simulink model "SIMULINK_U_f_C"  (R2018b)
settings: Solver=FixedStepAuto  StartTime=0.0  StopTime=sim_end_time  FixedStep=fixed_step_size  RelTol=1e-3
undefined symbols (not defined in the file): a, act_end, b, battery_threshold, bb, draw_gif, droneyeeUAV2_NUM, droneyeeUAV3_NUM, droneyeeUAV4_NUM, droneyeeUAV5_NUM, fixed_step_size, k, KD_x, KD_y, kd_z, KDD_x, KDD_y, KI_x, KI_y, ki_z, KII_x, KII_y, KP_x, KP_y, kp_z, KPP_x, KPP_y, lmt, omega, R, sim_end_time, uav10num, uav1num, uav2num, uav3num, uav4num, uav5num, uav6num, uav7num, uav8num, uav9num, UAV_NUM, Vel_Switch_1, Vel_Switch_10, Vel_Switch_11, Vel_Switch_12, Vel_Switch_13, Vel_Switch_14, Vel_Switch_15, Vel_Switch_16, Vel_Switch_17, Vel_Switch_18, Vel_Switch_19, Vel_Switch_2, Vel_Switch_20, Vel_Switch_3, Vel_Switch_4, Vel_Switch_5, Vel_Switch_6, Vel_Switch_7 ... (+11)
libraries: simulink x120, aerolibanimutils x1
(part 2 of 10)

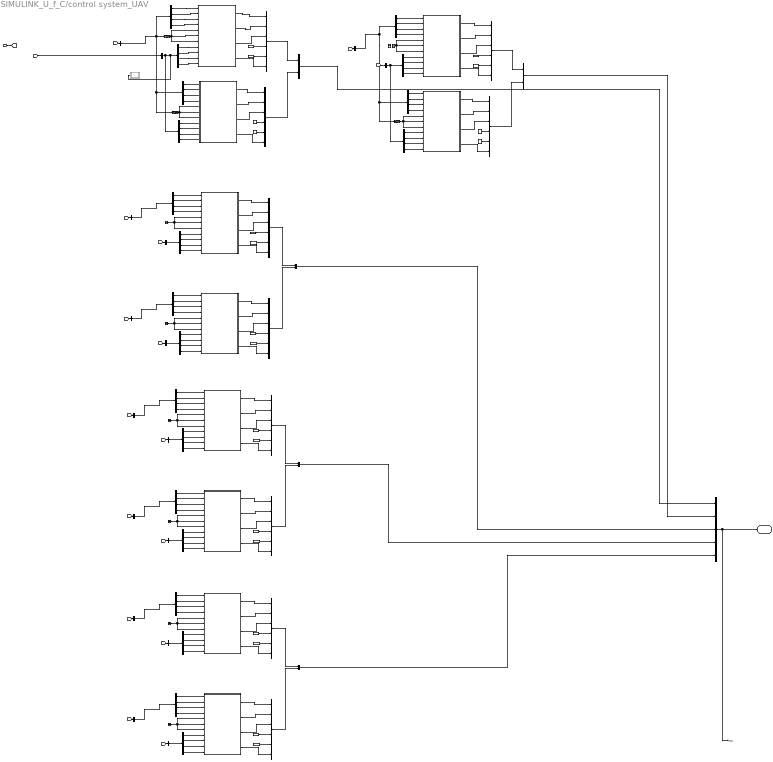
== system SIMULINK_U_f_C/control system_UAV ==
  uavstates_d : Inport
  Baseline Controller1 : Subsystem  AncestorBlock=ARBlocks/Baseline Controller
  Baseline Controller10 : Subsystem  AncestorBlock=ARBlocks/Baseline Controller
  Baseline Controller2 : Subsystem  AncestorBlock=ARBlocks/Baseline Controller
  Baseline Controller3 : Subsystem  AncestorBlock=ARBlocks/Baseline Controller
  Baseline Controller4 : Subsystem  AncestorBlock=ARBlocks/Baseline Controller
  Baseline Controller5 : Subsystem  AncestorBlock=ARBlocks/Baseline Controller
  Baseline Controller6 : Subsystem  AncestorBlock=ARBlocks/Baseline Controller
  Baseline Controller7 : Subsystem  AncestorBlock=ARBlocks/Baseline Controller
  Baseline Controller8 : Subsystem  AncestorBlock=ARBlocks/Baseline Controller
  Baseline Controller9 : Subsystem  AncestorBlock=ARBlocks/Baseline Controller
  Bus Creator{,1,3..4,6..7,9..10,12,14} (10 alike) : BusCreator  Inputs=6
  Bus Creator{2,5,8,11,13} (5 alike) : BusCreator  Inputs=2
  Bus Creator36 : BusCreator  Inputs=5
  Bus Selector : BusSelector  OutputSignals=droneyeeUAV1_states,droneyeeUAV2_states  OutputAsBus=on
  Bus Selector1 : BusSelector  OutputSignals=droneyeeUAV1_d.x1_d,droneyeeUAV1_d.y1_d,droneyeeUAV1_d.z1_d,droneyeeUAV1_d.yaw1_d
  Bus Selector10 : BusSelector  OutputSignals=droneyeeUAV4_d.x4_d,droneyeeUAV4_d.y4_d,droneyeeUAV4_d.z4_d,droneyeeUAV4_d.yaw4_d
  Bus Selector11 : BusSelector  OutputSignals=states_5_6_d
  Bus Selector12 : BusSelector  OutputSignals=droneyeeUAV3_states.x,droneyeeUAV3_states.y,droneyeeUAV3_states.z,droneyeeUAV3_states.yaw
  Bus Selector13 : BusSelector  OutputSignals=droneyeeUAV5_d.x5_d,droneyeeUAV5_d.y5_d,droneyeeUAV5_d.z5_d,droneyeeUAV5_d.yaw5_d
  Bus Selector14 : BusSelector  OutputSignals=states_7_8_d.droneyeeUAV8_d
  Bus Selector{15..16,24..25} (4 alike) : BusSelector  OutputSignals=x_d,y_d,z_d,yaw_d
  Bus Selector{6,17,20,23,26,29} (6 alike) : BusSelector  OutputSignals=x,y,z,yaw
  Bus Selector18 : BusSelector  OutputSignals=droneyeeUAV7_states
  Bus Selector19 : BusSelector  OutputSignals=states_7_8_d.droneyeeUAV7_d
  Bus Selector2 : BusSelector  OutputSignals=droneyeeUAV6_d.x_d,droneyeeUAV6_d.y_d,droneyeeUAV6_d.z_d,droneyeeUAV6_d.yaw_d
  Bus Selector21 : BusSelector  OutputSignals=droneyeeUAV8_states
  Bus Selector22 : BusSelector  OutputSignals=states_9_10_d.droneyeeUAV10_d
  Bus Selector27 : BusSelector  OutputSignals=droneyeeUAV9_states
  Bus Selector28 : BusSelector  OutputSignals=states_9_10_d.droneyeeUAV9_d
  Bus Selector3 : BusSelector  OutputSignals=droneyeeUAV2_states.x,droneyeeUAV2_states.y,droneyeeUAV2_states.z,droneyeeUAV2_states.yaw
  Bus Selector30 : BusSelector  OutputSignals=droneyeeUAV10_states
  Bus Selector31 : BusSelector  OutputSignals=droneyeeUAV3_states,droneyeeUAV4_states  OutputAsBus=on
  Bus Selector32 : BusSelector  OutputSignals=droneyeeUAV5_states
  Bus Selector37 : BusSelector  OutputSignals=states_5_6_d
  Bus Selector38 : BusSelector  OutputSignals=states1_2_d
  Bus Selector39 : BusSelector  OutputSignals=states_3_4_d
  Bus Selector4 : BusSelector  OutputSignals=droneyeeUAV2_d.x2_d,droneyeeUAV2_d.y2_d,droneyeeUAV2_d.z2_d,droneyeeUAV2_d.yaw2_d
  Bus Selector5 : BusSelector  OutputSignals=droneyeeUAV3_d.x3_d,droneyeeUAV3_d.y3_d,droneyeeUAV3_d.z3_d,droneyeeUAV3_d.yaw3_d
  Bus Selector7 : BusSelector  OutputSignals=droneyeeUAV6_states
  Bus Selector8 : BusSelector  OutputSignals=droneyeeUAV1_states.x,droneyeeUAV1_states.y,droneyeeUAV1_states.z,droneyeeUAV1_states.yaw
  Bus Selector9 : BusSelector  OutputSignals=droneyeeUAV4_states.x,droneyeeUAV4_states.y,droneyeeUAV4_states.z,droneyeeUAV4_states.yaw
  Constant{,1..19} (20 alike) : Constant  Value=0
  Goto : Goto  Commented=on  GotoTag=uav_ctrl  TagVisibility=global
  Ground{,1..9} (10 alike) : Ground
  MATLAB Function : MATLAB Function  Commented=on  TreatAsAtomicUnit=on
  Terminator{,1..3} (4 alike) : Terminator
  uav_ctrl : Outport
  tag scope: uav1_24_d=global
  wires:
  Bus Selector1/2 -> Baseline Controller1/9(y_d)  "<y1_d>"
  Bus Selector8/3 -> Baseline Controller1/3(" Z_e ")  "<z>"
  Bus Selector1/3 -> Baseline Controller1/10(Z_d)  "<z1_d>"
  Bus Selector8/4 -> Baseline Controller1/4(Yaw_e)  "<yaw>"
  Bus Selector3/4 -> Baseline Controller2/4(Yaw_e)  "<yaw>"
  Bus Selector3/2 -> Baseline Controller2/2(Y_e)  "<y>"
  Bus Selector1/1 -> Baseline Controller1/8(x_d)  "<x1_d>"
  Bus Selector3/1 -> Baseline Controller2/1(X_e)  "<x>"
  Ground2/1 -> Baseline Controller2/7("V_z "), Baseline Controller2/5(" V_x"), Baseline Controller2/6(V_y)
  Bus Selector8/1 -> Baseline Controller1/1(X_e)  "<x>"
  Bus Selector3/3 -> Baseline Controller2/3(" Z_e ")  "<z>"
  Bus Selector1/4 -> Baseline Controller1/11(Yaw_d)  "<yaw1_d>"
  Bus Selector8/2 -> Baseline Controller1/2(Y_e)  "<y>"
  Ground1/1 -> Baseline Controller1/5(" V_x"), Baseline Controller1/6(V_y), Baseline Controller1/7("V_z ")
  Baseline Controller1/1(ux) -> Bus Creator/1  "u_vx"
  Baseline Controller1/2(uy) -> Bus Creator/2  "u_vy"
  Baseline Controller1/3(Z_velocity_d. [-1,1]) -> Bus Creator/3  "u_vz"
  Baseline Controller1/4(yaw_rate_d [-1,1]) -> Bus Creator/6  "u_rate_yaw"
  Constant/1 -> Bus Creator/4  "u_rate_roll"
  Constant1/1 -> Bus Creator/5  "u_rate_pitch"
  Baseline Controller2/4(yaw_rate_d [-1,1]) -> Bus Creator1/6  "u_rate_yaw"
  Baseline Controller2/1(ux) -> Bus Creator1/1  "u_vx"
  Constant2/1 -> Bus Creator1/4  "u_rate_roll"
  Baseline Controller2/2(uy) -> Bus Creator1/2  "u_vy"
  Baseline Controller2/3(Z_velocity_d. [-1,1]) -> Bus Creator1/3  "u_vz"
  Constant3/1 -> Bus Creator1/5  "u_rate_pitch"
  Bus Creator/1 -> Bus Creator2/1  "uav1"
  Bus Creator1/1 -> Bus Creator2/2  "uav2"
  Bus Creator2/1 -> Bus Creator36/1  "ctrl_1_2"
  Bus Selector38/1 -> Bus Selector4/1, MATLAB Function/1(u), Bus Selector1/1  "<states1_2_d>"
  Bus Selector4/1 -> Baseline Controller2/8(x_d)  "<x2_d>"
  Bus Selector4/3 -> Baseline Controller2/10(Z_d)  "<z2_d>"
  Bus Selector4/2 -> Baseline Controller2/9(y_d)  "<y2_d>"
  Bus Selector4/4 -> Baseline Controller2/11(Yaw_d)  "<yaw2_d>"
  Ground/1 -> Baseline Controller4/7("V_z "), Baseline Controller4/5(" V_x"), Baseline Controller4/6(V_y)
  Bus Selector12/4 -> Baseline Controller3/4(Yaw_e)  "<yaw>"
  Constant4/1 -> Bus Creator3/4  "u_rate_roll"
  Baseline Controller4/3(Z_velocity_d. [-1,1]) -> Bus Creator4/3  "u_vz"
  Baseline Controller3/3(Z_velocity_d. [-1,1]) -> Bus Creator3/3  "u_vz"
  Bus Selector5/4 -> Baseline Controller3/11(Yaw_d)  "<yaw3_d>"
  Baseline Controller4/1(ux) -> Bus Creator4/1  "u_vx"
  Bus Selector10/1 -> Baseline Controller4/8(x_d)  "<x4_d>"
  Bus Selector12/2 -> Baseline Controller3/2(Y_e)  "<y>"
  Baseline Controller4/4(yaw_rate_d [-1,1]) -> Bus Creator4/6  "u_rate_yaw"
  Bus Selector5/3 -> Baseline Controller3/10(Z_d)  "<z3_d>"
  Ground3/1 -> Baseline Controller3/7("V_z "), Baseline Controller3/5(" V_x"), Baseline Controller3/6(V_y)
  Bus Selector12/1 -> Baseline Controller3/1(X_e)  "<x>"
  Bus Selector10/2 -> Baseline Controller4/9(y_d)  "<y4_d>"
  Bus Selector9/4 -> Baseline Controller4/4(Yaw_e)  "<yaw>"
  Bus Selector12/3 -> Baseline Controller3/3(" Z_e ")  "<z>"
  Baseline Controller4/2(uy) -> Bus Creator4/2  "u_vy"
  Constant7/1 -> Bus Creator4/5  "u_rate_pitch"
  Baseline Controller3/1(ux) -> Bus Creator3/1  "u_vx"
  Bus Selector9/1 -> Baseline Controller4/1(X_e)  "<x>"
  Bus Selector5/2 -> Baseline Controller3/9(y_d)  "<y3_d>"
  Bus Selector39/1 -> Bus Selector10/1, Bus Selector5/1  "<states_3_4_d>"
  Bus Selector10/4 -> Baseline Controller4/11(Yaw_d)  "<yaw4_d>"
  Constant5/1 -> Bus Creator3/5  "u_rate_pitch"
  Bus Selector5/1 -> Baseline Controller3/8(x_d)  "<x3_d>"
  Constant6/1 -> Bus Creator4/4  "u_rate_roll"
  Bus Creator5/1 -> Bus Creator36/2  "ctrl_3_4"
  Bus Selector10/3 -> Baseline Controller4/10(Z_d)  "<z4_d>"
  Bus Selector9/2 -> Baseline Controller4/2(Y_e)  "<y>"
  Bus Creator3/1 -> Bus Creator5/1  "uav3"
  Bus Selector9/3 -> Baseline Controller4/3(" Z_e ")  "<z>"
  Baseline Controller3/4(yaw_rate_d [-1,1]) -> Bus Creator3/6  "u_rate_yaw"
  Baseline Controller3/2(uy) -> Bus Creator3/2  "u_vy"
  Bus Creator4/1 -> Bus Creator5/2  "uav4"
  Bus Selector23/2 -> Baseline Controller5/2(Y_e)  "<y>"
  Baseline Controller5/1(ux) -> Bus Creator6/1  "u_vx"
  Bus Selector13/4 -> Baseline Controller5/11(Yaw_d)  "<yaw5_d>"
  Bus Selector37/1 -> Bus Selector13/1  "<states_5_6_d>"
  Bus Selector13/2 -> Baseline Controller5/9(y_d)  "<y5_d>"
  Bus Selector23/1 -> Baseline Controller5/1(X_e)  "<x>"
  Constant8/1 -> Bus Creator6/4  "u_rate_roll"
  Bus Selector23/3 -> Baseline Controller5/3(" Z_e ")  "<z>"
  Bus Selector13/3 -> Baseline Controller5/10(Z_d)  "<z5_d>"
  Bus Selector23/4 -> Baseline Controller5/4(Yaw_e)  "<yaw>"
  Ground4/1 -> Baseline Controller5/7("V_z "), Baseline Controller5/5(" V_x"), Baseline Controller5/6(V_y)
  Bus Creator8/1 -> Bus Creator36/3  "ctrl_5_6"
  Baseline Controller5/3(Z_velocity_d. [-1,1]) -> Bus Creator6/3  "u_vz"
  Constant9/1 -> Bus Creator6/5  "u_rate_pitch"
  Bus Selector13/1 -> Baseline Controller5/8(x_d)  "<x5_d>"
  Baseline Controller5/4(yaw_rate_d [-1,1]) -> Bus Creator6/6  "u_rate_yaw"
  Baseline Controller5/2(uy) -> Bus Creator6/2  "u_vy"
  Bus Selector31/1 -> Bus Selector12/1, Terminator/1, Bus Selector9/1
  Bus Selector32/1 -> Bus Selector23/1  "<droneyeeUAV5_states>"
  [uav_states] -> Bus Selector/1
  Bus Selector/1 -> Terminator1/1, Terminator2/1, Bus Selector3/1, Bus Selector8/1
  [uav_states] -> Bus Selector31/1
  [uav_states] -> Bus Selector32/1
  [uav1_24_d] -> Bus Selector37/1
  [uav1_24_d] -> Bus Selector38/1
  [uav1_24_d] -> Bus Selector39/1
  Bus Creator36/1 -> Goto/1, uav_ctrl/1
  uavstates_d/1 -> [uav1_24_d]
  Bus Selector2/2 -> Baseline Controller6/9(y_d)  "<y_d>"
  Bus Selector6/3 -> Baseline Controller6/3(" Z_e ")  "<z>"
  Baseline Controller6/4(yaw_rate_d [-1,1]) -> Bus Creator7/6  "u_rate_yaw"
  Constant11/1 -> Bus Creator7/5  "u_rate_pitch"
  Baseline Controller6/1(ux) -> Bus Creator7/1  "u_vx"
  Bus Selector2/4 -> Baseline Controller6/11(Yaw_d)  "<yaw_d>"
  Constant10/1 -> Bus Creator7/4  "u_rate_roll"
  Bus Selector6/2 -> Baseline Controller6/2(Y_e)  "<y>"
  Ground5/1 -> Baseline Controller6/7("V_z "), Baseline Controller6/5(" V_x"), Baseline Controller6/6(V_y)
  Bus Selector7/1 -> Bus Selector6/1  "<droneyeeUAV6_states>"
  Bus Selector6/1 -> Baseline Controller6/1(X_e)  "<x>"
  Bus Selector2/1 -> Baseline Controller6/8(x_d)  "<x_d>"
  Baseline Controller6/2(uy) -> Bus Creator7/2  "u_vy"
  Bus Selector6/4 -> Baseline Controller6/4(Yaw_e)  "<yaw>"
  [uav1_24_d] -> Bus Selector11/1
  Bus Selector11/1 -> Bus Selector2/1  "<states_5_6_d>"
  Baseline Controller6/3(Z_velocity_d. [-1,1]) -> Bus Creator7/3  "u_vz"
  Bus Selector2/3 -> Baseline Controller6/10(Z_d)  "<z_d>"
  [uav_states] -> Bus Selector7/1
  Bus Creator6/1 -> Bus Creator8/1  "ctrl_5"
  Bus Creator7/1 -> Bus Creator8/2  "ctrl_5"
  Bus Selector15/2 -> Baseline Controller7/9(y_d)  "<y_d>"
  [uav_states] -> Bus Selector21/1
  Baseline Controller8/2(uy) -> Bus Creator10/2  "u_vy"
  Bus Selector21/1 -> Bus Selector20/1  "<droneyeeUAV8_states>"
  Bus Selector14/1 -> Bus Selector16/1  "<droneyeeUAV8_d>"
  Bus Selector16/1 -> Baseline Controller8/8(x_d)  "<x_d>"
  Bus Selector20/2 -> Baseline Controller8/2(Y_e)  "<y>"
  Bus Selector20/1 -> Baseline Controller8/1(X_e)  "<x>"
  Ground7/1 -> Baseline Controller8/7("V_z "), Baseline Controller8/5(" V_x"), Baseline Controller8/6(V_y)
  Bus Selector16/4 -> Baseline Controller8/11(Yaw_d)  "<yaw_d>"
  Constant13/1 -> Bus Creator10/5  "u_rate_pitch"
  Bus Selector20/4 -> Baseline Controller8/4(Yaw_e)  "<yaw>"
  Baseline Controller8/4(yaw_rate_d [-1,1]) -> Bus Creator10/6  "u_rate_yaw"
  Bus Selector17/3 -> Baseline Controller7/3(" Z_e ")  "<z>"
  Bus Selector16/2 -> Baseline Controller8/9(y_d)  "<y_d>"
  Baseline Controller7/4(yaw_rate_d [-1,1]) -> Bus Creator9/6  "u_rate_yaw"
  Constant15/1 -> Bus Creator9/5  "u_rate_pitch"
  Bus Selector20/3 -> Baseline Controller8/3(" Z_e ")  "<z>"
  Bus Selector16/3 -> Baseline Controller8/10(Z_d)  "<z_d>"
  Baseline Controller7/1(ux) -> Bus Creator9/1  "u_vx"
  Bus Selector15/4 -> Baseline Controller7/11(Yaw_d)  "<yaw_d>"
  Constant14/1 -> Bus Creator9/4  "u_rate_roll"
  Baseline Controller8/3(Z_velocity_d. [-1,1]) -> Bus Creator10/3  "u_vz"
  Baseline Controller8/1(ux) -> Bus Creator10/1  "u_vx"
  Bus Selector17/2 -> Baseline Controller7/2(Y_e)  "<y>"
  Ground6/1 -> Baseline Controller7/7("V_z "), Baseline Controller7/5(" V_x"), Baseline Controller7/6(V_y)
  Bus Selector18/1 -> Bus Selector17/1  "<droneyeeUAV7_states>"
  Bus Selector17/1 -> Baseline Controller7/1(X_e)  "<x>"
  Bus Selector15/1 -> Baseline Controller7/8(x_d)  "<x_d>"
  Baseline Controller7/2(uy) -> Bus Creator9/2  "u_vy"
  Bus Creator10/1 -> Bus Creator11/2  "ctrl_5"
  Bus Selector17/4 -> Baseline Controller7/4(Yaw_e)  "<yaw>"
  Constant12/1 -> Bus Creator10/4  "u_rate_roll"
  [uav1_24_d] -> Bus Selector19/1
  [uav1_24_d] -> Bus Selector14/1
  Bus Selector19/1 -> Bus Selector15/1  "<droneyeeUAV7_d>"
  Baseline Controller7/3(Z_velocity_d. [-1,1]) -> Bus Creator9/3  "u_vz"
  Bus Selector15/3 -> Baseline Controller7/10(Z_d)  "<z_d>"
  [uav_states] -> Bus Selector18/1
  Bus Creator9/1 -> Bus Creator11/1  "ctrl_5"
  Bus Creator11/1 -> Bus Creator36/4  "ctrl_7_8"
  Bus Creator12/1 -> Bus Creator13/2  "ctrl_5"
  Bus Selector26/1 -> Baseline Controller9/1(X_e)  "<x>"
  Bus Selector24/1 -> Baseline Controller9/8(x_d)  "<x_d>"
  Bus Selector27/1 -> Bus Selector26/1  "<droneyeeUAV9_states>"
  Ground8/1 -> Baseline Controller9/7("V_z "), Baseline Controller9/5(" V_x"), Baseline Controller9/6(V_y)
  Baseline Controller10/1(ux) -> Bus Creator12/1  "u_vx"
  Baseline Controller9/2(uy) -> Bus Creator14/2  "u_vy"
  Bus Selector25/3 -> Baseline Controller10/10(Z_d)  "<z_d>"
  Bus Selector24/4 -> Baseline Controller9/11(Yaw_d)  "<yaw_d>"
  Constant18/1 -> Bus Creator14/4  "u_rate_roll"
  Bus Selector29/3 -> Baseline Controller10/3(" Z_e ")  "<z>"
  Baseline Controller9/4(yaw_rate_d [-1,1]) -> Bus Creator14/6  "u_rate_yaw"
  Constant19/1 -> Bus Creator14/5  "u_rate_pitch"
  Bus Selector26/3 -> Baseline Controller9/3(" Z_e ")  "<z>"
  Bus Selector25/2 -> Baseline Controller10/9(y_d)  "<y_d>"
  Baseline Controller10/4(yaw_rate_d [-1,1]) -> Bus Creator12/6  "u_rate_yaw"
  Bus Selector29/4 -> Baseline Controller10/4(Yaw_e)  "<yaw>"
  Ground9/1 -> Baseline Controller10/7("V_z "), Baseline Controller10/5(" V_x"), Baseline Controller10/6(V_y)
  Bus Selector25/4 -> Baseline Controller10/11(Yaw_d)  "<yaw_d>"
  Bus Selector29/1 -> Baseline Controller10/1(X_e)  "<x>"
  Baseline Controller10/3(Z_velocity_d. [-1,1]) -> Bus Creator12/3  "u_vz"
  Bus Selector29/2 -> Baseline Controller10/2(Y_e)  "<y>"
  Bus Selector25/1 -> Baseline Controller10/8(x_d)  "<x_d>"
  Bus Selector30/1 -> Bus Selector29/1  "<droneyeeUAV10_states>"
  Bus Selector22/1 -> Bus Selector25/1  "<droneyeeUAV10_d>"
  [uav_states] -> Bus Selector30/1
  Baseline Controller10/2(uy) -> Bus Creator12/2  "u_vy"
  Bus Selector24/2 -> Baseline Controller9/9(y_d)  "<y_d>"
  Bus Selector24/3 -> Baseline Controller9/10(Z_d)  "<z_d>"
  Bus Creator14/1 -> Bus Creator13/1  "ctrl_5"
  [uav1_24_d] -> Bus Selector28/1
  [uav_states] -> Bus Selector27/1
  Constant17/1 -> Bus Creator12/5  "u_rate_pitch"
  Bus Selector26/4 -> Baseline Controller9/4(Yaw_e)  "<yaw>"
  Bus Selector26/2 -> Baseline Controller9/2(Y_e)  "<y>"
  Constant16/1 -> Bus Creator12/4  "u_rate_roll"
  Baseline Controller9/3(Z_velocity_d. [-1,1]) -> Bus Creator14/3  "u_vz"
  [uav1_24_d] -> Bus Selector22/1
  Baseline Controller9/1(ux) -> Bus Creator14/1  "u_vx"
  Bus Selector28/1 -> Bus Selector24/1  "<droneyeeUAV9_d>"
  Bus Creator13/1 -> Bus Creator36/5  "ctrl_9_10"

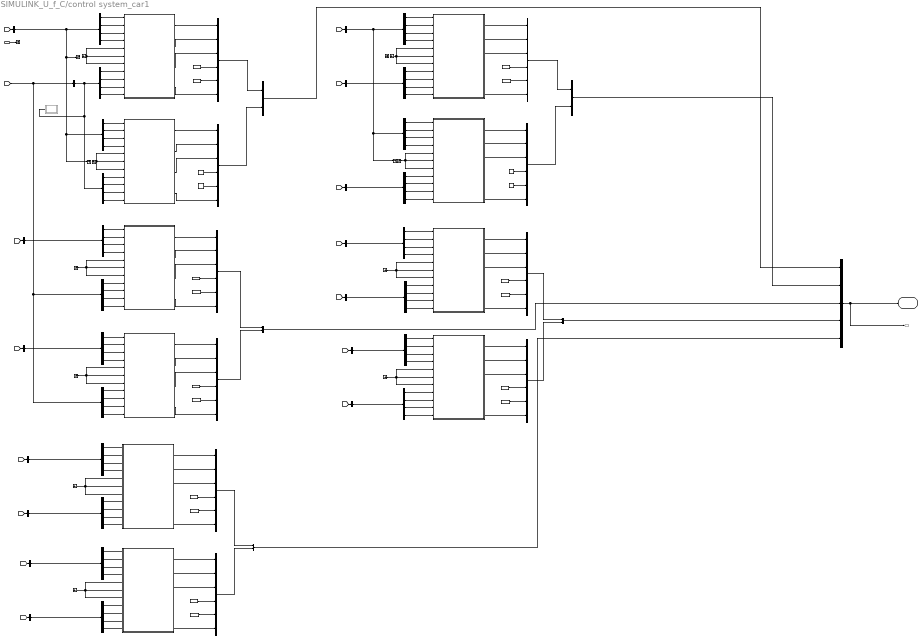
== system SIMULINK_U_f_C/control system_car1 ==
  CAR1-10_d : Inport
  Baseline Controller1 : Subsystem  AncestorBlock=ARBlocks/Baseline Controller
  Baseline Controller10 : Subsystem  AncestorBlock=ARBlocks/Baseline Controller
  Baseline Controller2 : Subsystem  AncestorBlock=ARBlocks/Baseline Controller
  Baseline Controller3 : Subsystem  AncestorBlock=ARBlocks/Baseline Controller
  Baseline Controller4 : Subsystem  AncestorBlock=ARBlocks/Baseline Controller
  Baseline Controller5 : Subsystem  AncestorBlock=ARBlocks/Baseline Controller
  Baseline Controller6 : Subsystem  AncestorBlock=ARBlocks/Baseline Controller
  Baseline Controller7 : Subsystem  AncestorBlock=ARBlocks/Baseline Controller
  Baseline Controller8 : Subsystem  AncestorBlock=ARBlocks/Baseline Controller
  Baseline Controller9 : Subsystem  AncestorBlock=ARBlocks/Baseline Controller
  Bus Creator{,1,3..4,6..7,9..10,12,14} (10 alike) : BusCreator  Inputs=6
  Bus Creator{2,5,8,11,13} (5 alike) : BusCreator  Inputs=2
  Bus Creator36 : BusCreator  Inputs=5
  Bus Selector : BusSelector  OutputSignals=droneyeeCAR1_states,droneyeeCAR2_states  OutputAsBus=on
  Bus Selector1 : BusSelector  OutputSignals=droneyeeCAR1_d.x1_d,droneyeeCAR1_d.y1_d,droneyeeCAR1_d.z1_d,droneyeeCAR1_d.yaw1_d
  Bus Selector10 : BusSelector  OutputSignals=x4_d,y4_d,z4_d,yaw4_d
  Bus Selector11 : BusSelector  OutputSignals=statesCAR3_4_d.droneyeeCAR3_d,statesCAR3_4_d.droneyeeCAR4_d  OutputAsBus=on
  Bus Selector12 : BusSelector  OutputSignals=droneyeeCAR3_states.x,droneyeeCAR3_states.y,droneyeeCAR3_states.z,droneyeeCAR3_states.yaw
  Bus Selector13 : BusSelector  OutputSignals=statesCAR5_6_d.droneyeeCAR5_d.x5_d,statesCAR5_6_d.droneyeeCAR5_d.y5_d,statesCAR5_6_d.droneyeeCAR5_d.z5_d,statesCAR5_6_d.droneyeeCAR5_d.yaw5_d
  Bus Selector14 : BusSelector  OutputSignals=statesCAR7_8_d.droneyeeCAR8_d  OutputAsBus=on
  Bus Selector15 : BusSelector  OutputSignals=x5_d,y5_d,z5_d,yaw5_d
  Bus Selector16 : BusSelector  OutputSignals=x1_d,y1_d,z1_d,yaw1_d
  Bus Selector{6,17,20,23,26,29} (6 alike) : BusSelector  OutputSignals=x,y,z,yaw
  Bus Selector18 : BusSelector  OutputSignals=droneyeeCAR7_states
  Bus Selector19 : BusSelector  OutputSignals=statesCAR7_8_d.droneyeeCAR7_d  OutputAsBus=on
  Bus Selector2 : BusSelector  OutputSignals=statesCAR5_6_d.droneyeeCAR6_d.x1_d,statesCAR5_6_d.droneyeeCAR6_d.y1_d,statesCAR5_6_d.droneyeeCAR6_d.z1_d,statesCAR5_6_d.droneyeeCAR6_d.yaw1_d
  Bus Selector21 : BusSelector  OutputSignals=droneyeeCAR8_states
  Bus Selector22 : BusSelector  OutputSignals=statesCAR9_10_d.droneyeeCAR10_d  OutputAsBus=on
  Bus Selector24 : BusSelector  OutputSignals=x5_d,y5_d,z5_d,yaw5_d
  Bus Selector25 : BusSelector  OutputSignals=x1_d,y1_d,z1_d,yaw1_d
  Bus Selector27 : BusSelector  OutputSignals=droneyeeCAR9_states
  Bus Selector28 : BusSelector  OutputSignals=statesCAR9_10_d.droneyeeCAR9_d  OutputAsBus=on
  Bus Selector3 : BusSelector  OutputSignals=droneyeeCAR2_states.x,droneyeeCAR2_states.y,droneyeeCAR2_states.z,droneyeeCAR2_states.yaw
  Bus Selector30 : BusSelector  OutputSignals=droneyeeCAR10_states
  Bus Selector31 : BusSelector  OutputSignals=droneyeeCAR3_states,droneyeeCAR4_states  OutputAsBus=on
  Bus Selector32 : BusSelector  OutputSignals=droneyeeCAR5_states
  Bus Selector33 : BusSelector  OutputSignals=statesCAR3_4_d.droneyeeCAR4_d  OutputAsBus=on
  Bus Selector38 : BusSelector  OutputSignals=statesCAR1_2_d
  Bus Selector4 : BusSelector  OutputSignals=droneyeeCAR2_d.x2_d,droneyeeCAR2_d.y2_d,droneyeeCAR2_d.z2_d,droneyeeCAR2_d.yaw2_d
  Bus Selector5 : BusSelector  OutputSignals=droneyeeCAR3_d.x3_d,droneyeeCAR3_d.y3_d,droneyeeCAR3_d.z3_d,droneyeeCAR3_d.yaw3_d
  Bus Selector7 : BusSelector  OutputSignals=droneyeeCAR6_states
  Bus Selector8 : BusSelector  OutputSignals=droneyeeCAR1_states.x,droneyeeCAR1_states.y,droneyeeCAR1_states.z,droneyeeCAR1_states.yaw
  Bus Selector9 : BusSelector  OutputSignals=droneyeeCAR4_states.x,droneyeeCAR4_states.y,droneyeeCAR4_states.z,droneyeeCAR4_states.yaw
  Constant{,1..19} (20 alike) : Constant  Value=0
  Goto : Goto  Commented=on  GotoTag=uav_ctrl  TagVisibility=global
  Ground{,1..9} (10 alike) : Ground
  MATLAB Function : MATLAB Function  Commented=on  TreatAsAtomicUnit=on
  Terminator{,1..4} (5 alike) : Terminator
  uav_ctrl : Outport
  wires:
  Bus Selector1/2 -> Baseline Controller1/9(y_d)  "<y1_d>"
  Bus Selector8/3 -> Baseline Controller1/3(" Z_e ")  "<z>"
  Bus Selector1/3 -> Baseline Controller1/10(Z_d)  "<z1_d>"
  Bus Selector8/4 -> Baseline Controller1/4(Yaw_e)  "<yaw>"
  Bus Selector3/4 -> Baseline Controller2/4(Yaw_e)  "<yaw>"
  Bus Selector3/2 -> Baseline Controller2/2(Y_e)  "<y>"
  Bus Selector1/1 -> Baseline Controller1/8(x_d)  "<x1_d>"
  Bus Selector3/1 -> Baseline Controller2/1(X_e)  "<x>"
  Ground2/1 -> Baseline Controller2/7("V_z "), Baseline Controller2/5(" V_x"), Baseline Controller2/6(V_y)
  Bus Selector8/1 -> Baseline Controller1/1(X_e)  "<x>"
  Bus Selector3/3 -> Baseline Controller2/3(" Z_e ")  "<z>"
  Bus Selector1/4 -> Baseline Controller1/11(Yaw_d)  "<yaw1_d>"
  Bus Selector8/2 -> Baseline Controller1/2(Y_e)  "<y>"
  Ground1/1 -> Baseline Controller1/7("V_z "), Baseline Controller1/5(" V_x"), Baseline Controller1/6(V_y)
  Baseline Controller1/1(ux) -> Bus Creator/1  "u_vx"
  Baseline Controller1/2(uy) -> Bus Creator/2  "u_vy"
  Baseline Controller1/3(Z_velocity_d. [-1,1]) -> Bus Creator/3  "u_vz"
  Baseline Controller1/4(yaw_rate_d [-1,1]) -> Bus Creator/6  "u_rate_yaw"
  Constant/1 -> Bus Creator/4  "u_rate_roll"
  Constant1/1 -> Bus Creator/5  "u_rate_pitch"
  Baseline Controller2/4(yaw_rate_d [-1,1]) -> Bus Creator1/6  "u_rate_yaw"
  Baseline Controller2/1(ux) -> Bus Creator1/1  "u_vx"
  Constant2/1 -> Bus Creator1/4  "u_rate_roll"
  Baseline Controller2/2(uy) -> Bus Creator1/2  "u_vy"
  Baseline Controller2/3(Z_velocity_d. [-1,1]) -> Bus Creator1/3  "u_vz"
  Constant3/1 -> Bus Creator1/5  "u_rate_pitch"
  Bus Creator/1 -> Bus Creator2/1  "CAR1"
  Bus Creator1/1 -> Bus Creator2/2  "CAR2"
  Bus Creator2/1 -> Bus Creator36/1  "ctrlCAR1_2"
  Bus Selector38/1 -> Bus Selector4/1, MATLAB Function/1(u), Bus Selector1/1  "<statesCAR1_2_d>"
  Bus Selector4/1 -> Baseline Controller2/8(x_d)  "<x2_d>"
  Bus Selector4/3 -> Baseline Controller2/10(Z_d)  "<z2_d>"
  Bus Selector4/2 -> Baseline Controller2/9(y_d)  "<y2_d>"
  Bus Selector4/4 -> Baseline Controller2/11(Yaw_d)  "<yaw2_d>"
  Ground/1 -> Baseline Controller4/5(" V_x"), Baseline Controller4/6(V_y), Baseline Controller4/7("V_z ")
  Bus Selector12/4 -> Baseline Controller3/4(Yaw_e)  "<yaw>"
  Constant4/1 -> Bus Creator3/4  "u_rate_roll"
  Baseline Controller4/3(Z_velocity_d. [-1,1]) -> Bus Creator4/3  "u_vz"
  Baseline Controller3/3(Z_velocity_d. [-1,1]) -> Bus Creator3/3  "u_vz"
  Bus Selector5/4 -> Baseline Controller3/11(Yaw_d)  "<yaw3_d>"
  Baseline Controller4/1(ux) -> Bus Creator4/1  "u_vx"
  Bus Selector10/1 -> Baseline Controller4/8(x_d)  "<x4_d>"
  Bus Selector12/2 -> Baseline Controller3/2(Y_e)  "<y>"
  Baseline Controller4/4(yaw_rate_d [-1,1]) -> Bus Creator4/6  "u_rate_yaw"
  Bus Selector5/3 -> Baseline Controller3/10(Z_d)  "<z3_d>"
  Ground3/1 -> Baseline Controller3/6(V_y), Baseline Controller3/5(" V_x"), Baseline Controller3/7("V_z ")
  Bus Selector12/1 -> Baseline Controller3/1(X_e)  "<x>"
  Bus Selector10/2 -> Baseline Controller4/9(y_d)  "<y4_d>"
  Bus Selector9/4 -> Baseline Controller4/4(Yaw_e)  "<yaw>"
  Bus Selector12/3 -> Baseline Controller3/3(" Z_e ")  "<z>"
  Baseline Controller4/2(uy) -> Bus Creator4/2  "u_vy"
  Constant7/1 -> Bus Creator4/5  "u_rate_pitch"
  Baseline Controller3/1(ux) -> Bus Creator3/1  "u_vx"
  Bus Selector9/1 -> Baseline Controller4/1(X_e)  "<x>"
  Bus Selector5/2 -> Baseline Controller3/9(y_d)  "<y3_d>"
  Bus Selector10/4 -> Baseline Controller4/11(Yaw_d)  "<yaw4_d>"
  Constant5/1 -> Bus Creator3/5  "u_rate_pitch"
  Bus Selector5/1 -> Baseline Controller3/8(x_d)  "<x3_d>"
  Constant6/1 -> Bus Creator4/4  "u_rate_roll"
  Bus Creator5/1 -> Bus Creator36/2  "ctrlCAR3_4"
  Bus Selector10/3 -> Baseline Controller4/10(Z_d)  "<z4_d>"
  Bus Selector9/2 -> Baseline Controller4/2(Y_e)  "<y>"
  Bus Creator3/1 -> Bus Creator5/1  "CAR3"
  Bus Selector9/3 -> Baseline Controller4/3(" Z_e ")  "<z>"
  Baseline Controller3/4(yaw_rate_d [-1,1]) -> Bus Creator3/6  "u_rate_yaw"
  Baseline Controller3/2(uy) -> Bus Creator3/2  "u_vy"
  Bus Creator4/1 -> Bus Creator5/2  "CAR4"
  Bus Selector23/2 -> Baseline Controller5/2(Y_e)  "<y>"
  Baseline Controller5/1(ux) -> Bus Creator6/1  "u_vx"
  Bus Selector13/4 -> Baseline Controller5/11(Yaw_d)  "<yaw5_d>"
  Bus Selector13/2 -> Baseline Controller5/9(y_d)  "<y5_d>"
  Bus Selector23/1 -> Baseline Controller5/1(X_e)  "<x>"
  Constant8/1 -> Bus Creator6/4  "u_rate_roll"
  Bus Selector23/3 -> Baseline Controller5/3(" Z_e ")  "<z>"
  Bus Selector13/3 -> Baseline Controller5/10(Z_d)  "<z5_d>"
  Bus Selector23/4 -> Baseline Controller5/4(Yaw_e)  "<yaw>"
  Ground4/1 -> Baseline Controller5/5(" V_x"), Baseline Controller5/7("V_z "), Baseline Controller5/6(V_y)
  Bus Creator8/1 -> Bus Creator36/3  "ctrlCAR5_6"
  Baseline Controller5/3(Z_velocity_d. [-1,1]) -> Bus Creator6/3  "u_vz"
  Constant9/1 -> Bus Creator6/5  "u_rate_pitch"
  Bus Selector13/1 -> Baseline Controller5/8(x_d)  "<x5_d>"
  Baseline Controller5/4(yaw_rate_d [-1,1]) -> Bus Creator6/6  "u_rate_yaw"
  Baseline Controller5/2(uy) -> Bus Creator6/2  "u_vy"
  Bus Selector31/1 -> Terminator/1, Bus Selector9/1, Bus Selector12/1
  Bus Selector32/1 -> Bus Selector23/1  "<droneyeeCAR5_states>"
  [uav_states] -> Bus Selector/1
  Bus Selector/1 -> Terminator1/1, Bus Selector3/1, Terminator2/1, Bus Selector8/1
  [uav_states] -> Bus Selector31/1
  [uav_states] -> Bus Selector32/1
  [car1_10_d] -> Bus Selector2/1, Bus Selector13/1, Bus Selector38/1
  Bus Creator36/1 -> Goto/1, uav_ctrl/1
  CAR1-10_d/1 -> Terminator4/1
  Bus Selector2/2 -> Baseline Controller6/9(y_d)  "<y1_d>"
  Bus Selector6/3 -> Baseline Controller6/3(" Z_e ")  "<z>"
  Baseline Controller6/4(yaw_rate_d [-1,1]) -> Bus Creator7/6  "u_rate_yaw"
  Constant11/1 -> Bus Creator7/5  "u_rate_pitch"
  Baseline Controller6/1(ux) -> Bus Creator7/1  "u_vx"
  Bus Selector2/4 -> Baseline Controller6/11(Yaw_d)  "<yaw1_d>"
  Constant10/1 -> Bus Creator7/4  "u_rate_roll"
  Bus Selector6/2 -> Baseline Controller6/2(Y_e)  "<y>"
  Ground5/1 -> Baseline Controller6/6(V_y), Baseline Controller6/5(" V_x"), Baseline Controller6/7("V_z ")
  Bus Selector7/1 -> Bus Selector6/1  "<droneyeeCAR6_states>"
  Bus Selector6/1 -> Baseline Controller6/1(X_e)  "<x>"
  Bus Selector2/1 -> Baseline Controller6/8(x_d)  "<x1_d>"
  Baseline Controller6/2(uy) -> Bus Creator7/2  "u_vy"
  Bus Selector6/4 -> Baseline Controller6/4(Yaw_e)  "<yaw>"
  Baseline Controller6/3(Z_velocity_d. [-1,1]) -> Bus Creator7/3  "u_vz"
  Bus Selector2/3 -> Baseline Controller6/10(Z_d)  "<z1_d>"
  [uav_states] -> Bus Selector7/1
  Bus Creator6/1 -> Bus Creator8/1  "CAR5"
  Bus Creator7/1 -> Bus Creator8/2  "CAR6"
  Bus Selector15/2 -> Baseline Controller7/9(y_d)  "<y5_d>"
  [uav_states] -> Bus Selector21/1
  Baseline Controller8/2(uy) -> Bus Creator10/2  "u_vy"
  Bus Selector21/1 -> Bus Selector20/1  "<droneyeeCAR8_states>"
  Bus Selector16/1 -> Baseline Controller8/8(x_d)  "<x1_d>"
  Bus Selector20/2 -> Baseline Controller8/2(Y_e)  "<y>"
  Bus Selector20/1 -> Baseline Controller8/1(X_e)  "<x>"
  Ground7/1 -> Baseline Controller8/5(" V_x"), Baseline Controller8/6(V_y), Baseline Controller8/7("V_z ")
  Bus Selector16/4 -> Baseline Controller8/11(Yaw_d)  "<yaw1_d>"
  Constant13/1 -> Bus Creator10/5  "u_rate_pitch"
  Bus Selector20/4 -> Baseline Controller8/4(Yaw_e)  "<yaw>"
  Baseline Controller8/4(yaw_rate_d [-1,1]) -> Bus Creator10/6  "u_rate_yaw"
  Bus Selector17/3 -> Baseline Controller7/3(" Z_e ")  "<z>"
  Bus Selector16/2 -> Baseline Controller8/9(y_d)  "<y1_d>"
  Baseline Controller7/4(yaw_rate_d [-1,1]) -> Bus Creator9/6  "u_rate_yaw"
  Constant15/1 -> Bus Creator9/5  "u_rate_pitch"
  Bus Selector20/3 -> Baseline Controller8/3(" Z_e ")  "<z>"
  Bus Selector16/3 -> Baseline Controller8/10(Z_d)  "<z1_d>"
  Baseline Controller7/1(ux) -> Bus Creator9/1  "u_vx"
  Bus Selector15/4 -> Baseline Controller7/11(Yaw_d)  "<yaw5_d>"
  Constant14/1 -> Bus Creator9/4  "u_rate_roll"
  Baseline Controller8/3(Z_velocity_d. [-1,1]) -> Bus Creator10/3  "u_vz"
  Baseline Controller8/1(ux) -> Bus Creator10/1  "u_vx"
  Bus Selector17/2 -> Baseline Controller7/2(Y_e)  "<y>"
  Ground6/1 -> Baseline Controller7/7("V_z "), Baseline Controller7/5(" V_x"), Baseline Controller7/6(V_y)
  Bus Selector18/1 -> Bus Selector17/1  "<droneyeeCAR7_states>"
  Bus Selector17/1 -> Baseline Controller7/1(X_e)  "<x>"
  Bus Selector15/1 -> Baseline Controller7/8(x_d)  "<x5_d>"
  Baseline Controller7/2(uy) -> Bus Creator9/2  "u_vy"
  Bus Creator10/1 -> Bus Creator11/2  "CAR8"
  Bus Selector17/4 -> Baseline Controller7/4(Yaw_e)  "<yaw>"
  Constant12/1 -> Bus Creator10/4  "u_rate_roll"
  Baseline Controller7/3(Z_velocity_d. [-1,1]) -> Bus Creator9/3  "u_vz"
  Bus Selector15/3 -> Baseline Controller7/10(Z_d)  "<z5_d>"
  [uav_states] -> Bus Selector18/1
  Bus Creator9/1 -> Bus Creator11/1  "CAR7"
  Bus Creator11/1 -> Bus Creator36/4  "ctrlCAR7_8"
  Bus Creator12/1 -> Bus Creator13/2  "CAR10"
  Bus Selector26/1 -> Baseline Controller9/1(X_e)  "<x>"
  Bus Selector24/1 -> Baseline Controller9/8(x_d)  "<x5_d>"
  Bus Selector27/1 -> Bus Selector26/1  "<droneyeeCAR9_states>"
  Ground8/1 -> Baseline Controller9/7("V_z "), Baseline Controller9/6(V_y), Baseline Controller9/5(" V_x")
  Baseline Controller10/1(ux) -> Bus Creator12/1  "u_vx"
  Baseline Controller9/2(uy) -> Bus Creator14/2  "u_vy"
  Bus Selector25/3 -> Baseline Controller10/10(Z_d)  "<z1_d>"
  Bus Selector24/4 -> Baseline Controller9/11(Yaw_d)  "<yaw5_d>"
  Constant18/1 -> Bus Creator14/4  "u_rate_roll"
  Bus Selector29/3 -> Baseline Controller10/3(" Z_e ")  "<z>"
  Baseline Controller9/4(yaw_rate_d [-1,1]) -> Bus Creator14/6  "u_rate_yaw"
  Constant19/1 -> Bus Creator14/5  "u_rate_pitch"
  Bus Selector26/3 -> Baseline Controller9/3(" Z_e ")  "<z>"
  Bus Selector25/2 -> Baseline Controller10/9(y_d)  "<y1_d>"
  Baseline Controller10/4(yaw_rate_d [-1,1]) -> Bus Creator12/6  "u_rate_yaw"
  Bus Selector29/4 -> Baseline Controller10/4(Yaw_e)  "<yaw>"
  Ground9/1 -> Baseline Controller10/6(V_y), Baseline Controller10/7("V_z "), Baseline Controller10/5(" V_x")
  Bus Selector25/4 -> Baseline Controller10/11(Yaw_d)  "<yaw1_d>"
  Bus Selector29/1 -> Baseline Controller10/1(X_e)  "<x>"
  Baseline Controller10/3(Z_velocity_d. [-1,1]) -> Bus Creator12/3  "u_vz"
  Bus Selector29/2 -> Baseline Controller10/2(Y_e)  "<y>"
  Bus Selector25/1 -> Baseline Controller10/8(x_d)  "<x1_d>"
  Bus Selector30/1 -> Bus Selector29/1  "<droneyeeCAR10_states>"
  [uav_states] -> Bus Selector30/1
  Baseline Controller10/2(uy) -> Bus Creator12/2  "u_vy"
  Bus Selector24/2 -> Baseline Controller9/9(y_d)  "<y5_d>"
  Bus Selector24/3 -> Baseline Controller9/10(Z_d)  "<z5_d>"
  Bus Creator14/1 -> Bus Creator13/1  "CAR9"
  [uav_states] -> Bus Selector27/1
  Constant17/1 -> Bus Creator12/5  "u_rate_pitch"
  Bus Selector26/4 -> Baseline Controller9/4(Yaw_e)  "<yaw>"
  Bus Selector26/2 -> Baseline Controller9/2(Y_e)  "<y>"
  Constant16/1 -> Bus Creator12/4  "u_rate_roll"
  Baseline Controller9/3(Z_velocity_d. [-1,1]) -> Bus Creator14/3  "u_vz"
  Baseline Controller9/1(ux) -> Bus Creator14/1  "u_vx"
  Bus Creator13/1 -> Bus Creator36/5  "ctrlCAR9_10"
  [car1_10_d] -> Bus Selector11/1
  Bus Selector11/1 -> Bus Selector5/1
  [car1_10_d] -> Bus Selector33/1
  Bus Selector33/1 -> Bus Selector10/1
  [car1_10_d] -> Bus Selector19/1
  Bus Selector19/1 -> Bus Selector15/1
  [car1_10_d] -> Bus Selector14/1
  Bus Selector14/1 -> Bus Selector16/1
  [car1_10_d] -> Bus Selector28/1
  Bus Selector28/1 -> Bus Selector24/1
  Bus Selector22/1 -> Bus Selector25/1
  [car1_10_d] -> Bus Selector22/1
